simulink model "RC_clanek"  (R2022b)
settings: Solver=VariableStepAuto  StartTime=0.0  StopTime=100.0  RelTol=1e-3
settings Model: Creator=honza  LastModifiedBy=honza

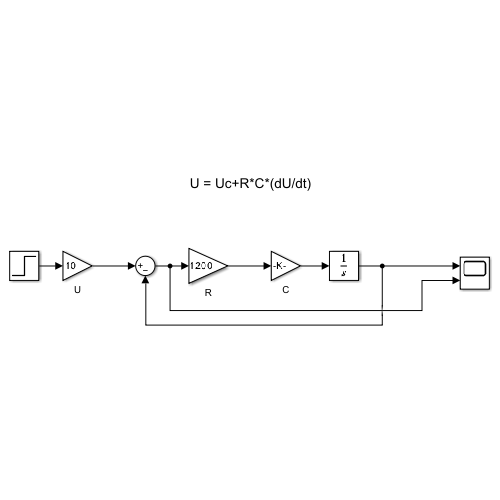
[thumbnail: Simulink's stored preview of the top-level diagram]
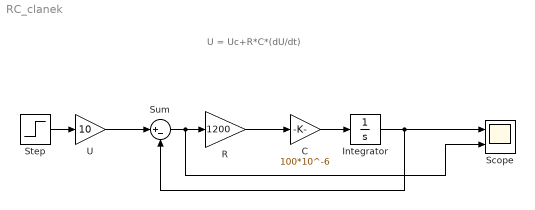
== system RC_clanek ==
  note: U = Uc+R*C*(dU/dt)
  C : Gain  Gain=100*10^-6
  Integrator : Integrator
  R : Gain  Gain=1200
  Scope : Scope  NumInputPorts=2
  Step : Step  Time=0  SampleTime=0
  Sum : Sum  Inputs=|+-
  U : Gain  Gain=10
  wires:
  Step/1 -> U/1
  R/1 -> C/1
  C/1 -> Integrator/1
  Sum/1 -> Scope/2, R/1
  U/1 -> Sum/1
  Integrator/1 -> Scope/1, Sum/2
